simulink model "new1"  (R2025a)
settings: Solver=ode15s  StartTime=0.0  StopTime=10.0  RelTol=1e-3
undefined symbols (not defined in the file): g, Rs, Rsl, Rw, Ry, ShaftDamping, SolverSampleTime
libraries: fl_lib x44, nesl_utility x13, ee_lib x12, slpidlib x3, spsThreePhaseParallelRLCBranchLib x1, simrfV2elements x1, eePwmGeneratorTwoLevel x1, simulink x1, spsabctodq0Lib x1, spspowerguiLib x1
settings Model: SimulationMode=accelerator  Creator=maska  LastModifiedBy=maska

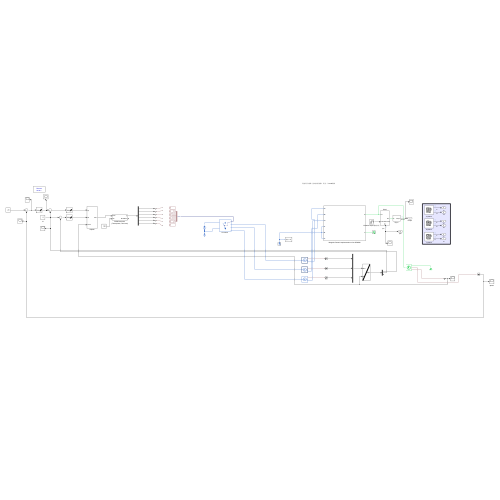
[thumbnail: Simulink's stored preview of the top-level diagram]
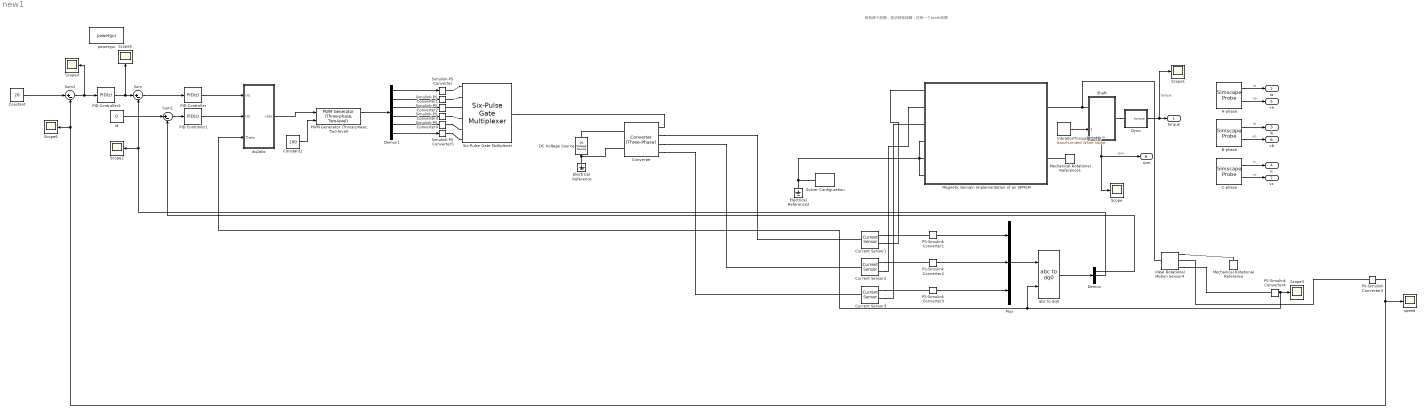
== system new1 ==
  note: 现有两个故障，扰动转矩故障，还有一个tooth故障
  A-phase : SimscapeProbe  BoundBlock=214  Variables="{\"i\":{\"Probing\":\"ON\"},\"n.v\":{\"Probing\":\"ON\"}}"
  B-phase : SimscapeProbe  BoundBlock=215  Variables="{\"i\":{\"Probing\":\"ON\"},\"n.v\":{\"Probing\":\"ON\"}}"
  C-phase : SimscapeProbe  BoundBlock=216  Variables="{\"i\":{\"Probing\":\"ON\"},\"n.v\":{\"Probing\":\"ON\"}}"
  Constant : Constant  Value=20
  Constant1 : Constant  Value=100
  Converter : ee_lib/Semiconductors & Converters/Converters/Converter (Three-Phase)  port_option=ee.enum.threePhasePort.expanded  fidelity_option=ee.enum.converters.fidelity.detailed  device_type=3  showThermalPort=false  K=0  Vth=0.5 V  Vgt=1 V  Vgt_off=-1 V  Ih=1 A  Vf=0.8 V  Ron=0.001 Ohm  Rds=0.001 Ohm  Goff=1e-5 1/Ohm  Eon_scalar=22.86e-3 J  Eoff_scalar=17.14e-3 J  Eoff_natural_commutation=10e-3 J  Voff=300 V  Iout_scalar=600 A  onCurrentMeasDelay=0 s  useCurrentFromPreviousCycle=false  useVoltageFromPreviousCycle=false  diode_param=2  diode_Vf=0.8 V  diode_Ron=0.001 Ohm  diode_Goff=1e-5 1/Ohm  diode_C=50 nF  diode_iRM=-235 A  diode_iF=300 A  diode_idot=-50 A/us  diode_trr_param=1  diode_trr_factor=3  diode_trr=15 us  diode_Qrr=1.5e+3 s*uA  diode_rec_loss_model=ee.enum.diode.reverseRecoveryModel.fixed  diode_ErecVal=0 J  diode_scaleWithIandV=false  diode_ErecMat=zeros(2, 3) J  diode_TjrecVec=[298.15, 398.15] K  diode_IfrecVec=[.1, 1, 10] A  diode_IrecVal=10 A  diode_VrecVal=10 V  diode_tFilter=1 / 1000 / 100 s  thermal_network_parameterization=ee.enum.thermalNetworkTopology.external  Rth=[.08, .5] K/W  Rth_Cauer=[.08, .1, .5] K/W  Rth_Foster=[.08, .14, .22, .16] K/W  thermal_mass_parameterization=ee.enum.thermalNetwork.timeconstant  thermal_mass=[.01, .5] J/K  thermal_mass_Cauer=[.01, .1, .5] J/K  thermal_mass_Foster=[.001, .005, .05, .5] J/K  thermal_time_constant=[.001, .2] s  thermal_time_constant_Cauer=[.001, .1, .2] s  thermal_time_constant_Foster=[7e-05, .0007, .01, .08] s  thermal_mass_initial_temperatures=[25, 25] degC  thermal_mass_initial_temperatures_Cauer=[25, 25, 25] degC  junction_thermal_mass=0.01 J/K  Tvec_initial_Foster=[25, 25, 25, 25] degC  snubber_type=0  Cs=1e-7 F  Rs=0.1 Ohm  Vce_loss=[0, 150, 300] V
      settings: InternalSimscapePortConfiguration="{\"Bottom\":[],\"Left\":[{\"id\":\"G\",\"label\":\"G\",\"type\":\"foundation.electrical.twelve_phase\"},{\"id\":\"a\",\"label\":\"a\",\"type\":\"foundation.electrical.electrical\"},{\"id\":\"b\",\"label\":\"b\",\"type\":\"foundation.electrical.electrical\"},{\"id\":\"c\",\"label\":\"c\",\"type\":\"foundation.electrical.electrical\"}],\"Right\":[{\"id\":\"p\",\"label\":\"+\",\"type\":\"foundation.electrical.electrical\"},{\"id\":\"n\",\"label\":\"-\",\"type\":\"foundation.electrical.electrical\"}],\"Top\":[]}"
  Current Sensor1 : fl_lib/Electrical/Electrical Sensors/Current Sensor
  Current Sensor2 : fl_lib/Electrical/Electrical Sensors/Current Sensor
  Current Sensor3 : fl_lib/Electrical/Electrical Sensors/Current Sensor
  DC Voltage Source : fl_lib/Electrical/Electrical Sources/DC Voltage Source  v0=750 V
  Demux : Demux  Outputs=3
  Demux1 : Demux  Outputs=6
  Dyno : Subsystem
  Electrical Reference : fl_lib/Electrical/Electrical Elements/Electrical Reference
  Electrical Reference2 : fl_lib/Electrical/Electrical Elements/Electrical Reference
  Ideal Rotational Motion Sensor4 : fl_lib/Mechanical/Mechanical Sensors/Ideal Rotational Motion Sensor  reference=foundation.enum.MeasurementReference.difference  acceleration_port=false  velocity_port=true  position_port=true  wrap_angle=false  offset=0 rad
  Magnetic Domain Implementation of an SPMSM : Subsystem
  Mechanical Rotational Reference : fl_lib/Mechanical/Rotational Elements/Mechanical Rotational Reference
  Mechanical Rotational Reference1 : fl_lib/Mechanical/Rotational Elements/Mechanical Rotational Reference
  Mux : Mux  Inputs=3
  PID Controller : slpidlib/PID Controller  Controller=PID  Form=Parallel  TimeDomain=Discrete-time  UseExternalTs=off  SampleTime=-1  IntegratorMethod=Forward Euler  FilterMethod=Forward Euler  ControllerParametersSource=internal  P=10  I=100  UseKiTs=off  D=0  UseExternalDerivativeSource=off  N=100  UseFilter=on  TunerSelectOption=Transfer Function Based (PID Tuner App)  InitialConditionSource=internal  InitialConditionForIntegrator=0  InitialConditionForFilter=0  DifferentiatorICPrevScaledInput=0  ExternalReset=none  TrackingMode=off  Kt=1  LimitOutput=on  SatLimitsSource=internal  UpperSaturationLimit=1000  LowerSaturationLimit=-1000  LinearizeAsGain=on  AntiWindupMode=none  Kb=1  LimitIntegrator=off  UpperIntegratorSaturationLimit=inf  LowerIntegratorSaturationLimit=-inf  POutMin=[]  POutMax=[]  IOutMin=[]  IOutMax=[]  DOutMin=[]  DOutMax=[]  NOutMin=[]  NOutMax=[]  SumOutMin=[]  SumOutMax=[]  SaturationOutMin=[]  SaturationOutMax=[]  PParamMin=[]  PParamMax=[]  IParamMin=[]  IParamMax=[]  DParamMin=[]  DParamMax=[]  NParamMin=[]  NParamMax=[]  KbParamMin=[]  KbParamMax=[]  KtParamMin=[]  KtParamMax=[]  KbOutMin=[]  KbOutMax=[]  KtOutMin=[]  KtOutMax=[]  IntegratorOutMin=[]  IntegratorOutMax=[]  FilterOutMin=[]  FilterOutMax=[]  SumI1OutMin=[]  SumI1OutMax=[]  SumI2OutMin=[]  SumI2OutMax=[]  SumI3OutMin=[]  SumI3OutMax=[]  SumI4OutMin=[]  SumI4OutMax=[]  SumDOutMin=[]  SumDOutMax=[]  DifferentiatorOutMin=[]  DifferentiatorOutMax=[]  FilterDiffOutCoefMin=[]  FilterDiffOutCoefMax=[]  ReciprocalOutMin=[]  ReciprocalOutMax=[]  SumDenOutMin=[]  SumDenOutMax=[]  SumNumOutMin=[]  SumNumOutMax=[]  DivideOutMin=[]  DivideOutMax=[]  UdiffTsProdOutMin=[]  UdiffTsProdOutMax=[]  NTsProdOutMin=[]  NTsProdOutMax=[]  UintegralTsProdOutMin=[]  UintegralTsProdOutMax=[]  UngainTsProdOutMin=[]  UngainTsProdOutMax=[]  ClampingZeroOutDataTypeStr=Inherit: Inherit via back propagation  ClampingZeroOutMin=[]  ClampingZeroOutMax=[]  FilterDenConstantOutDataTypeStr=Inherit: Inherit via back propagation  FilterDenConstantOutMin=[]  FilterDenConstantOutMax=[]  PCopyOutDataTypeStr=Inherit: Inherit via back propagation  PCopyOutMin=[]  PCopyOutMax=[]  NCopyOutDataTypeStr=Inherit: Inherit via back propagation  NCopyOutMin=[]  NCopyOutMax=[]  IntegratorContinuousStateAttributes=''  IntegratorStateMustResolveToSignalObject=off  IntegratorRTWStateStorageClass=Auto  FilterContinuousStateAttributes=''  FilterStateMustResolveToSignalObject=off  FilterRTWStateStorageClass=Auto  ParallelPVariant=InternalParameters  IdealPVariant=Disabled  IVariant=InternalParameters  DVariant=InternalParameters  IntegratorVariant=Discrete  SatVariant=Enabled  AWVariant=Passthrough  PCopyVariant=Disabled  TRVariant=Disabled  FdbkBlocksVariant=Forward  IdealPFdbkVariant=Disabled  SatFdbkVariant=Disabled  DerivativeFilterVariant=ForwardEulerFilter  NVariant=InternalParameters  NCopyVariant=Disabled  FilterICVariant=InternalICsFilter  IntegratorICVariant=InternalICs  ExternalResetVariant=Disabled  TRSumVariant=Passthrough  SumFdbkVariant=Disabled  SumVariant=Sum_PID  TsampFilterVariant=InternalTs  TsampNgainVariant=Passthrough  TsampIntegralVariant=Disabled_SignalSpec  ExternalSaturationOutDataTypeStr=Inherit: Same as second input  DerivativeSourceVariant=ErrorSignal  PreIntVariant=InternalPreInt
  PID Controller1 : slpidlib/PID Controller  Controller=PID  Form=Parallel  TimeDomain=Discrete-time  UseExternalTs=off  SampleTime=-1  IntegratorMethod=Forward Euler  FilterMethod=Forward Euler  ControllerParametersSource=internal  P=4  I=45  UseKiTs=off  D=0  UseExternalDerivativeSource=off  N=100  UseFilter=on  TunerSelectOption=Transfer Function Based (PID Tuner App)  InitialConditionSource=internal  InitialConditionForIntegrator=0  InitialConditionForFilter=0  DifferentiatorICPrevScaledInput=0  ExternalReset=none  TrackingMode=off  Kt=1  LimitOutput=on  SatLimitsSource=internal  UpperSaturationLimit=1000  LowerSaturationLimit=-1000  LinearizeAsGain=on  AntiWindupMode=none  Kb=1  LimitIntegrator=off  UpperIntegratorSaturationLimit=inf  LowerIntegratorSaturationLimit=-inf  POutMin=[]  POutMax=[]  IOutMin=[]  IOutMax=[]  DOutMin=[]  DOutMax=[]  NOutMin=[]  NOutMax=[]  SumOutMin=[]  SumOutMax=[]  SaturationOutMin=[]  SaturationOutMax=[]  PParamMin=[]  PParamMax=[]  IParamMin=[]  IParamMax=[]  DParamMin=[]  DParamMax=[]  NParamMin=[]  NParamMax=[]  KbParamMin=[]  KbParamMax=[]  KtParamMin=[]  KtParamMax=[]  KbOutMin=[]  KbOutMax=[]  KtOutMin=[]  KtOutMax=[]  IntegratorOutMin=[]  IntegratorOutMax=[]  FilterOutMin=[]  FilterOutMax=[]  SumI1OutMin=[]  SumI1OutMax=[]  SumI2OutMin=[]  SumI2OutMax=[]  SumI3OutMin=[]  SumI3OutMax=[]  SumI4OutMin=[]  SumI4OutMax=[]  SumDOutMin=[]  SumDOutMax=[]  DifferentiatorOutMin=[]  DifferentiatorOutMax=[]  FilterDiffOutCoefMin=[]  FilterDiffOutCoefMax=[]  ReciprocalOutMin=[]  ReciprocalOutMax=[]  SumDenOutMin=[]  SumDenOutMax=[]  SumNumOutMin=[]  SumNumOutMax=[]  DivideOutMin=[]  DivideOutMax=[]  UdiffTsProdOutMin=[]  UdiffTsProdOutMax=[]  NTsProdOutMin=[]  NTsProdOutMax=[]  UintegralTsProdOutMin=[]  UintegralTsProdOutMax=[]  UngainTsProdOutMin=[]  UngainTsProdOutMax=[]  ClampingZeroOutDataTypeStr=Inherit: Inherit via back propagation  ClampingZeroOutMin=[]  ClampingZeroOutMax=[]  FilterDenConstantOutDataTypeStr=Inherit: Inherit via back propagation  FilterDenConstantOutMin=[]  FilterDenConstantOutMax=[]  PCopyOutDataTypeStr=Inherit: Inherit via back propagation  PCopyOutMin=[]  PCopyOutMax=[]  NCopyOutDataTypeStr=Inherit: Inherit via back propagation  NCopyOutMin=[]  NCopyOutMax=[]  IntegratorContinuousStateAttributes=''  IntegratorStateMustResolveToSignalObject=off  IntegratorRTWStateStorageClass=Auto  FilterContinuousStateAttributes=''  FilterStateMustResolveToSignalObject=off  FilterRTWStateStorageClass=Auto  ParallelPVariant=InternalParameters  IdealPVariant=Disabled  IVariant=InternalParameters  DVariant=InternalParameters  IntegratorVariant=Discrete  SatVariant=Enabled  AWVariant=Passthrough  PCopyVariant=Disabled  TRVariant=Disabled  FdbkBlocksVariant=Forward  IdealPFdbkVariant=Disabled  SatFdbkVariant=Disabled  DerivativeFilterVariant=ForwardEulerFilter  NVariant=InternalParameters  NCopyVariant=Disabled  FilterICVariant=InternalICsFilter  IntegratorICVariant=InternalICs  ExternalResetVariant=Disabled  TRSumVariant=Passthrough  SumFdbkVariant=Disabled  SumVariant=Sum_PID  TsampFilterVariant=InternalTs  TsampNgainVariant=Passthrough  TsampIntegralVariant=Disabled_SignalSpec  ExternalSaturationOutDataTypeStr=Inherit: Same as second input  DerivativeSourceVariant=ErrorSignal  PreIntVariant=InternalPreInt
  PID Controller2 : slpidlib/PID Controller  Controller=PID  Form=Parallel  TimeDomain=Discrete-time  UseExternalTs=off  SampleTime=-1  IntegratorMethod=Forward Euler  FilterMethod=Forward Euler  ControllerParametersSource=internal  P=2.5  I=40  UseKiTs=off  D=0  UseExternalDerivativeSource=off  N=100  UseFilter=on  TunerSelectOption=Transfer Function Based (PID Tuner App)  InitialConditionSource=internal  InitialConditionForIntegrator=0  InitialConditionForFilter=0  DifferentiatorICPrevScaledInput=0  ExternalReset=none  TrackingMode=off  Kt=1  LimitOutput=on  SatLimitsSource=internal  UpperSaturationLimit=10000  LowerSaturationLimit=-10000  LinearizeAsGain=on  AntiWindupMode=none  Kb=1  LimitIntegrator=off  UpperIntegratorSaturationLimit=inf  LowerIntegratorSaturationLimit=-inf  POutMin=[]  POutMax=[]  IOutMin=[]  IOutMax=[]  DOutMin=[]  DOutMax=[]  NOutMin=[]  NOutMax=[]  SumOutMin=[]  SumOutMax=[]  SaturationOutMin=[]  SaturationOutMax=[]  PParamMin=[]  PParamMax=[]  IParamMin=[]  IParamMax=[]  DParamMin=[]  DParamMax=[]  NParamMin=[]  NParamMax=[]  KbParamMin=[]  KbParamMax=[]  KtParamMin=[]  KtParamMax=[]  KbOutMin=[]  KbOutMax=[]  KtOutMin=[]  KtOutMax=[]  IntegratorOutMin=[]  IntegratorOutMax=[]  FilterOutMin=[]  FilterOutMax=[]  SumI1OutMin=[]  SumI1OutMax=[]  SumI2OutMin=[]  SumI2OutMax=[]  SumI3OutMin=[]  SumI3OutMax=[]  SumI4OutMin=[]  SumI4OutMax=[]  SumDOutMin=[]  SumDOutMax=[]  DifferentiatorOutMin=[]  DifferentiatorOutMax=[]  FilterDiffOutCoefMin=[]  FilterDiffOutCoefMax=[]  ReciprocalOutMin=[]  ReciprocalOutMax=[]  SumDenOutMin=[]  SumDenOutMax=[]  SumNumOutMin=[]  SumNumOutMax=[]  DivideOutMin=[]  DivideOutMax=[]  UdiffTsProdOutMin=[]  UdiffTsProdOutMax=[]  NTsProdOutMin=[]  NTsProdOutMax=[]  UintegralTsProdOutMin=[]  UintegralTsProdOutMax=[]  UngainTsProdOutMin=[]  UngainTsProdOutMax=[]  ClampingZeroOutDataTypeStr=Inherit: Inherit via back propagation  ClampingZeroOutMin=[]  ClampingZeroOutMax=[]  FilterDenConstantOutDataTypeStr=Inherit: Inherit via back propagation  FilterDenConstantOutMin=[]  FilterDenConstantOutMax=[]  PCopyOutDataTypeStr=Inherit: Inherit via back propagation  PCopyOutMin=[]  PCopyOutMax=[]  NCopyOutDataTypeStr=Inherit: Inherit via back propagation  NCopyOutMin=[]  NCopyOutMax=[]  IntegratorContinuousStateAttributes=''  IntegratorStateMustResolveToSignalObject=off  IntegratorRTWStateStorageClass=Auto  FilterContinuousStateAttributes=''  FilterStateMustResolveToSignalObject=off  FilterRTWStateStorageClass=Auto  ParallelPVariant=InternalParameters  IdealPVariant=Disabled  IVariant=InternalParameters  DVariant=InternalParameters  IntegratorVariant=Discrete  SatVariant=Enabled  AWVariant=Passthrough  PCopyVariant=Disabled  TRVariant=Disabled  FdbkBlocksVariant=Forward  IdealPFdbkVariant=Disabled  SatFdbkVariant=Disabled  DerivativeFilterVariant=ForwardEulerFilter  NVariant=InternalParameters  NCopyVariant=Disabled  FilterICVariant=InternalICsFilter  IntegratorICVariant=InternalICs  ExternalResetVariant=Disabled  TRSumVariant=Passthrough  SumFdbkVariant=Disabled  SumVariant=Sum_PID  TsampFilterVariant=InternalTs  TsampNgainVariant=Passthrough  TsampIntegralVariant=Disabled_SignalSpec  ExternalSaturationOutDataTypeStr=Inherit: Same as second input  DerivativeSourceVariant=ErrorSignal  PreIntVariant=InternalPreInt
  PS-Simulink Converter{1..5} (5 alike) : nesl_utility/PS-Simulink Converter  PhysicalDomain=network_engine_domain  SubClassName=ps_output  LeftPortType=input  RightPortType=output  PseudoPeriodic=off  Frequencies=[]  VectorFormat=inherit  Unit=inherit  AffineConversion=off
  "PWM Generator (Three-phase, Two-level)" : eePwmGeneratorTwoLevel/PWM Generator (Three-phase, Two-level)  PWMMode=Continuous PWM (CPWM)  CPWMMode=SPWM: sinusoidal PWM  DPWMMode=60 DPWM: 60 degree discontinuous PWM  fsw=1e3  Ts=2e-6
      settings: LibrarySourceBlock=|
      | ee_sl_lib/Pulse Width
      | Modulation/PWM Generator
      | (Three-phase, Two-level)
  Scope{,1..6} (7 alike) : Scope
      Scope settings: ActiveDisplayYMinimum=5.9889874068411224  ActiveDisplayYMaximum=16.410945963930487
      Scope1 settings: ActiveDisplayYMinimum=-17672.734869868404  ActiveDisplayYMaximum=1963.7070418694955  DataLoggingVariableName=ScopeData2
      Scope2 settings: ActiveDisplayYMinimum=-0.416473738906253  ActiveDisplayYMaximum=0.436398147050316  YLabel=скорость  DataLoggingVariableName=ScopeData5
      Scope3 settings: ActiveDisplayYMinimum=-20.943872983065386  ActiveDisplayYMaximum=188.49485684758849  DataLoggingVariableName=ScopeData3
      Scope4 settings: ActiveDisplayYMinimum=2.2678285118136117  ActiveDisplayYMaximum=20.092232680750982  YLabel=скорость  DataLoggingVariableName=ScopeData8
      Scope5 settings: ActiveDisplayYMinimum=-203.76901912599916  ActiveDisplayYMaximum=1942.3454210939431  YLabel=скорость  DataLoggingVariableName=ScopeData9
      Scope6 settings: ActiveDisplayYMinimum=-2.0472362485662443  ActiveDisplayYMaximum=18.4251262370962  YLabel=скорость  DataLoggingVariableName=ScopeData6
  Shaft : Subsystem
      settings: PortSchema="{\"entries\":[{\"content\":{\"sides\":[{\"content\":{\"connectorIds\":[\"In1\",\"LConn1\"]},\"type\":\"ConnectorPlacement.EquallySpacedRectSide\",\"uuid\":\"d15f0b0a-376f-42bd-94fa-6b80795b7e9e\"},{\"content\":{\"connectorIds\":[\"RConn1\"],\"side\":\"RIGHT\"},\"type\":\"ConnectorPlacement.EquallySpacedRectSide\",\"uuid\":\"1c10d066-ee05-4c09-9add-16f0039017c8\"},{\"content\":{\"connectorIds\":[\"Out1\"],\"side\":\"TOP\"},\"type\":\"ConnectorPlacement.EquallySpacedRectSide\",\"uuid\":\"1eb1d482-04bc-4375-925a-bb39b5ad5755\"},{\"content\":{\"side\":\"BOTTOM\"},\"type\":\"ConnectorPlacement.EquallySpacedRectSide\",\"uuid\":\"41e2e734-a35c-40f7-83b7-7f9932e1f2da\"}]},\"type\":\"ConnectorPlacement.EquallySpacedConnector\",\"uuid\":\"850c0d3a-bd0e-4af5-8553-9696ca3cdee9\"}],\"packageUris\":[\"http://schema.mathworks.com/mf0/Connector/R2020b\"],\"version\":\"1.0\"}"
  Simulink-PS Converter{,1..5} (6 alike) : nesl_utility/Simulink-PS Converter  PhysicalDomain=network_engine_domain  SubClassName=ps_input  LeftPortType=input  RightPortType=output  PseudoPeriodic=off  Frequencies=[]  NoiseDistribution=none  NoiseParameters=[]  Unit=1  AffineConversion=off  FilteringAndDerivatives=provide  SimscapeFilterOrder=1  InputFilterTimeConstant=0.001  UdotUserProvided=0
  Six-Pulse Gate Multiplexer : ee_lib/Semiconductors & Converters/Converters/Six-Pulse Gate Multiplexer  port_option=ee.enum.controlport.ps
  Solver Configuration : nesl_utility/Solver Configuration  PhysicalDomain=network_engine_domain  SubClassName=solver  LeftPortType=input  RightPortType=generic  Tones=[]  Harmonics=[]  SimulateNoise=off  Profile=off  UseLocalSampling=off  EnableSwitchedLinearOptims=on  FrequencyDomain=off  UseCCode=off  RelTol=0.001  AbsTol=1e-06  MinStep=1e-09  ToWorkspace=off  RevertToSquareIcSolve=off  NumHomotopyIterations=100  PhasorMode=off  PhasorModeNumHarmonics=1  ConsistencySolver=NEWTON_FTOL  IndexReductionMethod=DerivativeReplacement  DoDC=off  ResidualTolerance=1e-09  ConsistencyTolSource=GLOBAL  ConsistencyAbsTol=0.001  ConsistencyRelTol=0.001  ConsistencyTolFactor=0.001  UseLocalSolver=on  LocalSolverChoice=NE_BACKWARD_EULER_ADVANCER  ResolveIndetEquations=on  FunctionEvalNumThread=1  LocalSolverSampleTime=SolverSampleTime  DoFixedCost=off  MaxNonlinIter=3  MaxModeIter=2  ComputeImpulses=off  ImpulseIterations=1  LinearAlgebra=auto  LinearAlgebraNumThread=0  EquationFormulation=NE_TIME_EF  DelaysMemoryBudget=1024  AutomaticFiltering=on  FilteringTimeConstant=0.001  PartitionStorageMethod=AS_NEEDED  PartitionMemoryBudget=1024  PartitionMethod=ROBUST  MultibodyUseLocalSolver=off  MultibodyLocalSolverChoice=ODE1  MultibodyLocalSolverSampleTime=0.001
  Sum : Sum  Inputs=|+-
  Sum1 : Sum  Inputs=|+-
  Sum2 : Sum  Inputs=|+-
  VibrationTorque震动转矩 : simulink/Sources/Band-Limited White Noise  Cov=VibrationNoisePower  Ts=SolverSampleTime  seed=[23341]
  abc to dq0 : spsabctodq0Lib/abc to dq0  Alignment=90 degrees behind phase A axis
  dq2abc : Subsystem
  id : Constant  Value=0
  powergui : spspowerguiLib/powergui  Priority=1  SimulationMode=Discrete  SampleTime=2e-6  frequency=60  Iterations=50  frequencyindice=0  Pbase=100e6  ErrMax=1e-4  UnitsV=kV  UnitsW=MW  buscounter=0  FunctionMessages=off  echomessages=off  EnableUseOfTLC=off  CurrentSourceSwitches=off  DisableSnubberDevices=off  DisableRonSwitches=off  DisableVfSwitches=off  DisplayEquations=off  AutomaticDiscreteSolvers=off  SolverType=Tustin/Backward Euler (TBE)  Interpol=off  ExternalGateDelay=off  methode=off  Ts=100  x0status=blocks  SPID=on  SwTol=0  HookPort=off  NonlinearTolerance=1e-4  nMaxIteration=100  ContinueOnMaxIteration=off  RestoreLinks=warning  ResistiveCurrentMeasurement=off  Frange=[0:2:500]  Ylog=off  Xlog=on  ShowGrid=off  save=off  variable=ZData  structure=0  ZoomFFT=off  StartTime=0.0  cycles=1  DisplayStyle=1  fundamental=60  FreqAxis=off  MaxFrequency=1000  frequencyindicesteady=1  RmsSteady=1  display=off
  speed : Scope
      settings: ActiveDisplayYMinimum=15.541713214540213  ActiveDisplayYMaximum=15.760330288068594  DataLoggingVariableName=ScopeData7
  torque : Outport
  ia : Outport  Port=2
  ib : Outport  Port=3
  ic : Outport  Port=4
  va : Outport  Port=5
  vb : Outport  Port=6
  vc : Outport  Port=7
  rpm : Outport  Port=8
  wires:
  VibrationTorque震动转矩/1 -> Shaft/1(PerturbationTorque)
  Dyno/1(torque) -> Scope1/1, torque/1  "torque"
  B-phase/2 -> vb/1  "vb"
  C-phase/2 -> vc/1  "vc"
  A-phase/1 -> ia/1  "ia"
  Shaft/1(rpm) -> Scope/1, rpm/1  "rpm"
  C-phase/1 -> ic/1  "ic"
  B-phase/1 -> ib/1  "ib"
  A-phase/2 -> va/1  "va"
  Sum2/1 -> Scope4/1, PID Controller2/1
  PID Controller2/1 -> Sum/1, Scope5/1
  Constant/1 -> Sum2/1
  id/1 -> Sum1/1
  Sum1/1 -> PID Controller1/1
  Demux/1 -> Sum1/2
  PS-Simulink Converter5/1 -> speed/1, Sum2/2, Scope6/1
  Demux/2 -> Scope2/1, Sum/2
  PS-Simulink Converter4/1 -> dq2abc/3(Theta), abc to dq0/2, Scope3/1
  PID Controller/1 -> dq2abc/1(Uq)
  PID Controller1/1 -> dq2abc/2(Ud)
  Sum/1 -> PID Controller/1
  PS-Simulink Converter3/1 -> Mux/3
  PS-Simulink Converter2/1 -> Mux/2
  PS-Simulink Converter1/1 -> Mux/1
  Mux/1 -> abc to dq0/1
  abc to dq0/1 -> Demux/1
  Constant1/1 -> "PWM Generator (Three-phase, Two-level)"/2
  dq2abc/1(vabc) -> "PWM Generator (Three-phase, Two-level)"/1
  "PWM Generator (Three-phase, Two-level)"/1 -> Demux1/1
  Demux1/6 -> Simulink-PS Converter5/1
  Demux1/5 -> Simulink-PS Converter4/1
  Demux1/2 -> Simulink-PS Converter1/1
  Demux1/1 -> Simulink-PS Converter/1
  Demux1/4 -> Simulink-PS Converter3/1
  Demux1/3 -> Simulink-PS Converter2/1
  connections:
  Solver Configuration/RConn1 -- Electrical Reference2/LConn1 -- Magnetic Domain Implementation of an SPMSM/LConn4 -- Magnetic Domain Implementation of an SPMSM/LConn5 -- Magnetic Domain Implementation of an SPMSM/LConn6
  Ideal Rotational Motion Sensor4/LConn1 -- Magnetic Domain Implementation of an SPMSM/RConn1 -- Shaft/LConn1
  Shaft/RConn1 -- Dyno/LConn1
  Electrical Reference/LConn1 -- Converter/RConn2 -- DC Voltage Source/RConn1
  DC Voltage Source/LConn1 -- Converter/RConn1
  Current Sensor3/RConn2 -- Magnetic Domain Implementation of an SPMSM/LConn3
  Current Sensor2/RConn2 -- Magnetic Domain Implementation of an SPMSM/LConn2
  Current Sensor1/RConn2 -- Magnetic Domain Implementation of an SPMSM/LConn1
  Converter/LConn2 -- Current Sensor1/LConn1
  Converter/LConn3 -- Current Sensor2/LConn1
  Converter/LConn4 -- Current Sensor3/LConn1
  Current Sensor1/RConn1 -- PS-Simulink Converter1/LConn1
  Current Sensor2/RConn1 -- PS-Simulink Converter2/LConn1
  Current Sensor3/RConn1 -- PS-Simulink Converter3/LConn1
  Mechanical Rotational Reference1/LConn1 -- Magnetic Domain Implementation of an SPMSM/RConn2
  Ideal Rotational Motion Sensor4/RConn1 -- Mechanical Rotational Reference/LConn1
  Ideal Rotational Motion Sensor4/RConn3 -- PS-Simulink Converter4/LConn1
  PS-Simulink Converter5/LConn1 -- Ideal Rotational Motion Sensor4/RConn2
  Simulink-PS Converter5/RConn1 -- Six-Pulse Gate Multiplexer/LConn6
  Simulink-PS Converter3/RConn1 -- Six-Pulse Gate Multiplexer/LConn4
  Simulink-PS Converter/RConn1 -- Six-Pulse Gate Multiplexer/LConn1
  Simulink-PS Converter4/RConn1 -- Six-Pulse Gate Multiplexer/LConn5
  Simulink-PS Converter2/RConn1 -- Six-Pulse Gate Multiplexer/LConn3
  Simulink-PS Converter1/RConn1 -- Six-Pulse Gate Multiplexer/LConn2
  Six-Pulse Gate Multiplexer/RConn1 -- Converter/LConn1

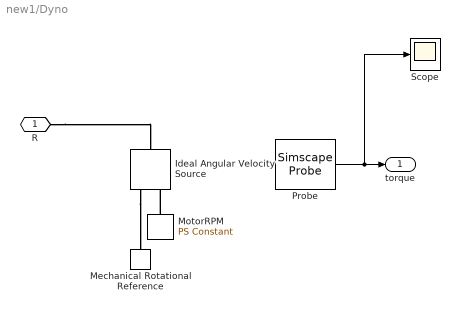
== system new1/Dyno ==
  Ideal Angular Velocity Source : fl_lib/Mechanical/Mechanical Sources/Ideal Angular Velocity Source
  Mechanical Rotational Reference : fl_lib/Mechanical/Rotational Elements/Mechanical Rotational Reference
  MotorRPM : fl_lib/Physical Signals/Sources/PS Constant  constant=motorRPM rpm
  Probe : SimscapeProbe  BoundBlock=148  Variables="{\"t\":{\"Probing\":\"ON\"}}"
  Scope : Scope
      settings: ActiveDisplayYMinimum=-17672.741352339104  ActiveDisplayYMaximum=1963.7653841058097
  R : PMIOPort  Side=Left
  torque : Outport
  wires:
  Probe/1 -> Scope/1, torque/1
  connections:
  MotorRPM/RConn1 -- Ideal Angular Velocity Source/RConn1
  Ideal Angular Velocity Source/RConn2 -- Mechanical Rotational Reference/LConn1
  R/RConn1 -- Ideal Angular Velocity Source/LConn1

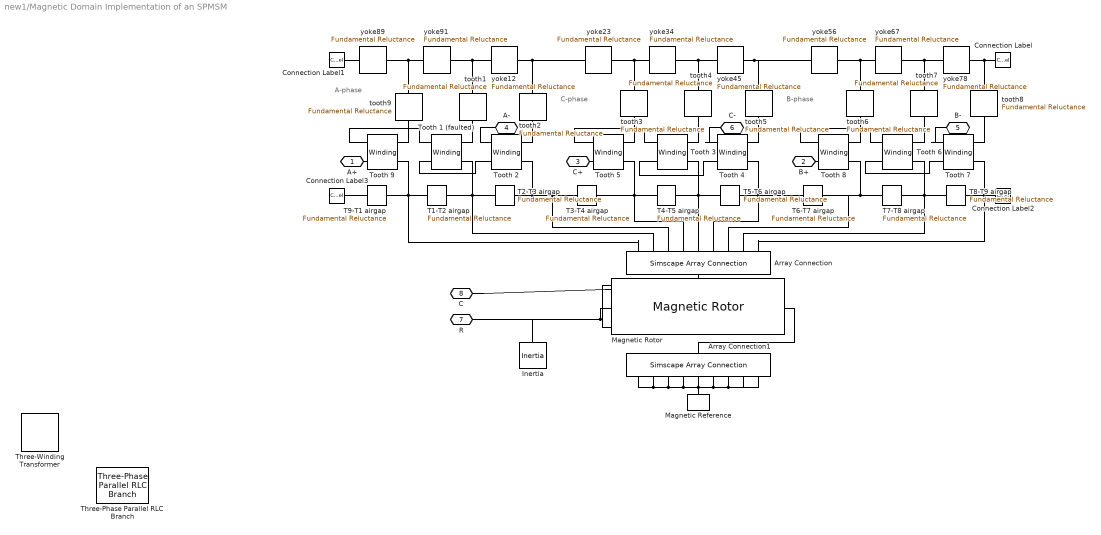
== system new1/Magnetic Domain Implementation of an SPMSM ==
  note: A-phase
  note: C-phase
  note: B-phase
  Array Connection : SimscapeArrayConnection  Domain=foundation.magnetic.magnetic  NumScalarElements=9
  Array Connection1 : SimscapeArrayConnection  Domain=foundation.magnetic.magnetic  NumScalarElements=9
  Connection Label : ConnectionLabel  Label=Y
  Connection Label1 : ConnectionLabel  Label=Y
  Connection Label2 : ConnectionLabel  Label=SL
  Connection Label3 : ConnectionLabel  Label=SL
  Inertia : fl_lib/Mechanical/Rotational Elements/Inertia  inertia=J kg*m^2  num_ports=foundation.enum.numPorts2.one  w_specify=on  w_priority=None  w=0 rad/s  w_nominal_specify=off  w_nominal_value=1  w_nominal_unit=rad/s  t_specify=off  t_priority=High  t=0 N*m  t_nominal_specify=off  t_nominal_value=1  t_nominal_unit=N*m
  Magnetic Reference : fl_lib/Magnetic/Magnetic Elements/Magnetic Reference
      settings: InternalSimscapePortConfiguration="{\"Bottom\":[],\"Left\":[{\"id\":\"M\",\"label\":\"\",\"type\":\"foundation.magnetic.magnetic\"}],\"Right\":[],\"Top\":[]}"
  Magnetic Rotor : ee_lib/Electromechanical/Magnetic Rotor  Nr=Npp  Ns=Ns  B0=B0 T  lm=lm mm  mur=1.05  g=g mm  r=r mm  l=l mm
      settings: InternalSimscapePortConfiguration="{\"Bottom\":[{\"id\":\"S\",\"label\":\"S\",\"type\":\"foundation.magnetic.magnetic\"}],\"Left\":[{\"id\":\"C\",\"label\":\"C\",\"type\":\"foundation.mechanical.rotational.rotational\"},{\"id\":\"R\",\"label\":\"R\",\"type\":\"foundation.mechanical.rotational.rotational\"}],\"Right\":[],\"Top\":[{\"id\":\"N\",\"label\":\"N\",\"type\":\"foundation.magnetic.magnetic\"}]}"
  T1-T2 airgap : fl_lib/Magnetic/Magnetic Elements/Fundamental Reluctance  R=Rsl 1/H  phi_specify=off  phi_priority=None  phi=0 Wb  phi_nominal_specify=off  phi_nominal_value=1  phi_nominal_unit=Wb  mmf_specify=off  mmf_priority=None  mmf=0 A  mmf_nominal_specify=off  mmf_nominal_value=1  mmf_nominal_unit=A
      settings: InternalSimscapePortConfiguration="{\"Bottom\":[],\"Left\":[{\"id\":\"N\",\"label\":\"N\",\"type\":\"foundation.magnetic.magnetic\"}],\"Right\":[{\"id\":\"S\",\"label\":\"S\",\"type\":\"foundation.magnetic.magnetic\"}],\"Top\":[]}"
  T2-T3 airgap : fl_lib/Magnetic/Magnetic Elements/Fundamental Reluctance  R=Rsl 1/H  phi_specify=off  phi_priority=None  phi=0 Wb  phi_nominal_specify=off  phi_nominal_value=1  phi_nominal_unit=Wb  mmf_specify=off  mmf_priority=None  mmf=0 A  mmf_nominal_specify=off  mmf_nominal_value=1  mmf_nominal_unit=A
      settings: InternalSimscapePortConfiguration="{\"Bottom\":[],\"Left\":[{\"id\":\"N\",\"label\":\"N\",\"type\":\"foundation.magnetic.magnetic\"}],\"Right\":[{\"id\":\"S\",\"label\":\"S\",\"type\":\"foundation.magnetic.magnetic\"}],\"Top\":[]}"
  T3-T4 airgap : fl_lib/Magnetic/Magnetic Elements/Fundamental Reluctance  R=Rsl 1/H  phi_specify=off  phi_priority=None  phi=0 Wb  phi_nominal_specify=off  phi_nominal_value=1  phi_nominal_unit=Wb  mmf_specify=off  mmf_priority=None  mmf=0 A  mmf_nominal_specify=off  mmf_nominal_value=1  mmf_nominal_unit=A
      settings: InternalSimscapePortConfiguration="{\"Bottom\":[],\"Left\":[{\"id\":\"N\",\"label\":\"N\",\"type\":\"foundation.magnetic.magnetic\"}],\"Right\":[{\"id\":\"S\",\"label\":\"S\",\"type\":\"foundation.magnetic.magnetic\"}],\"Top\":[]}"
  T4-T5 airgap : fl_lib/Magnetic/Magnetic Elements/Fundamental Reluctance  R=Rsl 1/H  phi_specify=off  phi_priority=None  phi=0 Wb  phi_nominal_specify=off  phi_nominal_value=1  phi_nominal_unit=Wb  mmf_specify=off  mmf_priority=None  mmf=0 A  mmf_nominal_specify=off  mmf_nominal_value=1  mmf_nominal_unit=A
      settings: InternalSimscapePortConfiguration="{\"Bottom\":[],\"Left\":[{\"id\":\"N\",\"label\":\"N\",\"type\":\"foundation.magnetic.magnetic\"}],\"Right\":[{\"id\":\"S\",\"label\":\"S\",\"type\":\"foundation.magnetic.magnetic\"}],\"Top\":[]}"
  T5-T6 airgap : fl_lib/Magnetic/Magnetic Elements/Fundamental Reluctance  R=Rsl 1/H  phi_specify=off  phi_priority=None  phi=0 Wb  phi_nominal_specify=off  phi_nominal_value=1  phi_nominal_unit=Wb  mmf_specify=off  mmf_priority=None  mmf=0 A  mmf_nominal_specify=off  mmf_nominal_value=1  mmf_nominal_unit=A
      settings: InternalSimscapePortConfiguration="{\"Bottom\":[],\"Left\":[{\"id\":\"N\",\"label\":\"N\",\"type\":\"foundation.magnetic.magnetic\"}],\"Right\":[{\"id\":\"S\",\"label\":\"S\",\"type\":\"foundation.magnetic.magnetic\"}],\"Top\":[]}"
  T6-T7 airgap : fl_lib/Magnetic/Magnetic Elements/Fundamental Reluctance  R=Rsl 1/H  phi_specify=off  phi_priority=None  phi=0 Wb  phi_nominal_specify=off  phi_nominal_value=1  phi_nominal_unit=Wb  mmf_specify=off  mmf_priority=None  mmf=0 A  mmf_nominal_specify=off  mmf_nominal_value=1  mmf_nominal_unit=A
      settings: InternalSimscapePortConfiguration="{\"Bottom\":[],\"Left\":[{\"id\":\"N\",\"label\":\"N\",\"type\":\"foundation.magnetic.magnetic\"}],\"Right\":[{\"id\":\"S\",\"label\":\"S\",\"type\":\"foundation.magnetic.magnetic\"}],\"Top\":[]}"
  T7-T8 airgap : fl_lib/Magnetic/Magnetic Elements/Fundamental Reluctance  R=Rsl 1/H  phi_specify=off  phi_priority=None  phi=0 Wb  phi_nominal_specify=off  phi_nominal_value=1  phi_nominal_unit=Wb  mmf_specify=off  mmf_priority=None  mmf=0 A  mmf_nominal_specify=off  mmf_nominal_value=1  mmf_nominal_unit=A
      settings: InternalSimscapePortConfiguration="{\"Bottom\":[],\"Left\":[{\"id\":\"N\",\"label\":\"N\",\"type\":\"foundation.magnetic.magnetic\"}],\"Right\":[{\"id\":\"S\",\"label\":\"S\",\"type\":\"foundation.magnetic.magnetic\"}],\"Top\":[]}"
  T8-T9 airgap : fl_lib/Magnetic/Magnetic Elements/Fundamental Reluctance  R=Rsl 1/H  phi_specify=off  phi_priority=None  phi=0 Wb  phi_nominal_specify=off  phi_nominal_value=1  phi_nominal_unit=Wb  mmf_specify=off  mmf_priority=None  mmf=0 A  mmf_nominal_specify=off  mmf_nominal_value=1  mmf_nominal_unit=A
      settings: InternalSimscapePortConfiguration="{\"Bottom\":[],\"Left\":[{\"id\":\"N\",\"label\":\"N\",\"type\":\"foundation.magnetic.magnetic\"}],\"Right\":[{\"id\":\"S\",\"label\":\"S\",\"type\":\"foundation.magnetic.magnetic\"}],\"Top\":[]}"
  T9-T1 airgap : fl_lib/Magnetic/Magnetic Elements/Fundamental Reluctance  R=Rsl 1/H  phi_specify=off  phi_priority=None  phi=0 Wb  phi_nominal_specify=off  phi_nominal_value=1  phi_nominal_unit=Wb  mmf_specify=off  mmf_priority=None  mmf=0 A  mmf_nominal_specify=off  mmf_nominal_value=1  mmf_nominal_unit=A
      settings: InternalSimscapePortConfiguration="{\"Bottom\":[],\"Left\":[{\"id\":\"N\",\"label\":\"N\",\"type\":\"foundation.magnetic.magnetic\"}],\"Right\":[{\"id\":\"S\",\"label\":\"S\",\"type\":\"foundation.magnetic.magnetic\"}],\"Top\":[]}"
  Three-Phase Parallel RLC Branch : spsThreePhaseParallelRLCBranchLib/Three-Phase Parallel RLC Branch  LConnTagsString=A|B|C  RConnTagsString=A|B|C  BranchType=RLC  Resistance=1  Inductance=1e-3  Capacitance=1e-6  Measurements=None
  Three-Winding Transformer : simrfV2elements/Three-Winding Transformer  classname=three_winding_transformer  L1=1e-6 H  L2=1e-6 H  L3=1e-6 H  K12=0.9  K13=0.9  K23=0.9
  Tooth 1 (faulted) : ee_lib/Passive/Winding  Nw=Nws  Rw=Rw/3 Ohm  Rl=inf 1/H  Gw=gWinding 1/Ohm  thermalPort=simscape.enum.thermaleffects.omit  alpha=3.93e-3 1/K  Tmeas=25 degC  winding_thermal_mass=100 J/K  T_specify=off  T_priority=None  T=25 degC  T_nominal_specify=off  T_nominal_value=1  T_nominal_unit=degC  i_specify=off  i_priority=None  i=0 A  i_nominal_specify=off  i_nominal_value=1  i_nominal_unit=A  v_specify=off  v_priority=High  v=0 V  v_nominal_specify=off  v_nominal_value=1  v_nominal_unit=V  phi_specify=off  phi_priority=None  phi=0 Wb  phi_nominal_specify=off  phi_nominal_value=1  phi_nominal_unit=Wb  iterm_p_specify=off  iterm_p_priority=None  iterm_p=0 A  iterm_p_nominal_specify=off  iterm_p_nominal_value=1  iterm_p_nominal_unit=A  iterm_n_specify=off  iterm_n_priority=None  iterm_n=0 A  iterm_n_nominal_specify=off  iterm_n_nominal_value=1  iterm_n_nominal_unit=A  power_dissipated_specify=off  power_dissipated_priority=None  power_dissipated=0 W  power_dissipated_nominal_specify=off  power_dissipated_nominal_value=1  power_dissipated_nominal_unit=W
      settings: InternalSimscapePortConfiguration="{\"Bottom\":[],\"Left\":[{\"id\":\"p\",\"label\":\"+\",\"type\":\"foundation.electrical.electrical\"},{\"id\":\"n\",\"label\":\"-\",\"type\":\"foundation.electrical.electrical\"}],\"Right\":[{\"id\":\"N\",\"label\":\"N\",\"type\":\"foundation.magnetic.magnetic\"},{\"id\":\"S\",\"label\":\"S\",\"type\":\"foundation.magnetic.magnetic\"}],\"Top\":[]}"
  Tooth {2..9} (8 alike) : ee_lib/Passive/Winding  Nw=Nws  Rw=Rw/3 Ohm  Rl=inf 1/H  Gw=gWinding 1/Ohm  thermalPort=simscape.enum.thermaleffects.omit  alpha=3.93e-3 1/K  Tmeas=25 degC  winding_thermal_mass=100 J/K  T_specify=off  T_priority=None  T=25 degC  T_nominal_specify=off  T_nominal_value=1  T_nominal_unit=degC  i_specify=off  i_priority=None  i=0 A  i_nominal_specify=off  i_nominal_value=1  i_nominal_unit=A  v_specify=off  v_priority=None  v=0 V  v_nominal_specify=off  v_nominal_value=1  v_nominal_unit=V  phi_specify=off  phi_priority=None  phi=0 Wb  phi_nominal_specify=off  phi_nominal_value=1  phi_nominal_unit=Wb  iterm_p_specify=off  iterm_p_priority=None  iterm_p=0 A  iterm_p_nominal_specify=off  iterm_p_nominal_value=1  iterm_p_nominal_unit=A  iterm_n_specify=off  iterm_n_priority=None  iterm_n=0 A  iterm_n_nominal_specify=off  iterm_n_nominal_value=1  iterm_n_nominal_unit=A  power_dissipated_specify=off  power_dissipated_priority=None  power_dissipated=0 W  power_dissipated_nominal_specify=off  power_dissipated_nominal_value=1  power_dissipated_nominal_unit=W
      settings: InternalSimscapePortConfiguration="{\"Bottom\":[],\"Left\":[{\"id\":\"p\",\"label\":\"+\",\"type\":\"foundation.electrical.electrical\"},{\"id\":\"n\",\"label\":\"-\",\"type\":\"foundation.electrical.electrical\"}],\"Right\":[{\"id\":\"N\",\"label\":\"N\",\"type\":\"foundation.magnetic.magnetic\"},{\"id\":\"S\",\"label\":\"S\",\"type\":\"foundation.magnetic.magnetic\"}],\"Top\":[]}"
  tooth{1..9} (9 alike) : fl_lib/Magnetic/Magnetic Elements/Fundamental Reluctance  R=Rs 1/H  phi_specify=off  phi_priority=None  phi=0 Wb  phi_nominal_specify=off  phi_nominal_value=1  phi_nominal_unit=Wb  mmf_specify=off  mmf_priority=None  mmf=0 A  mmf_nominal_specify=off  mmf_nominal_value=1  mmf_nominal_unit=A
      settings: InternalSimscapePortConfiguration="{\"Bottom\":[],\"Left\":[{\"id\":\"N\",\"label\":\"N\",\"type\":\"foundation.magnetic.magnetic\"}],\"Right\":[{\"id\":\"S\",\"label\":\"S\",\"type\":\"foundation.magnetic.magnetic\"}],\"Top\":[]}"
  yoke{12,23,34,45,56,67,78,89,91} (9 alike) : fl_lib/Magnetic/Magnetic Elements/Fundamental Reluctance  R=Ry 1/H  phi_specify=off  phi_priority=None  phi=0 Wb  phi_nominal_specify=off  phi_nominal_value=1  phi_nominal_unit=Wb  mmf_specify=off  mmf_priority=None  mmf=0 A  mmf_nominal_specify=off  mmf_nominal_value=1  mmf_nominal_unit=A
      settings: InternalSimscapePortConfiguration="{\"Bottom\":[],\"Left\":[{\"id\":\"N\",\"label\":\"N\",\"type\":\"foundation.magnetic.magnetic\"}],\"Right\":[{\"id\":\"S\",\"label\":\"S\",\"type\":\"foundation.magnetic.magnetic\"}],\"Top\":[]}"
  A+ : PMIOPort  Side=Left
  B+ : PMIOPort  Port=2  Side=Left
  C+ : PMIOPort  Port=3  Side=Left
  A- : PMIOPort  Port=4  Side=Left
  B- : PMIOPort  Port=5  Side=Left
  C- : PMIOPort  Port=6  Side=Left
  R : PMIOPort  Port=7  Side=Right
  C : PMIOPort  Port=8  Side=Right
  connections:
  yoke91/RConn1 -- yoke12/LConn1 -- tooth1/LConn1
  Tooth 1 (faulted)/RConn2 -- Array Connection/LConn2 -- T2-T3 airgap/LConn1 -- T1-T2 airgap/RConn1
  T3-T4 airgap/LConn1 -- Array Connection/LConn3 -- Tooth 2/RConn2 -- T2-T3 airgap/RConn1
  Tooth 2/RConn1 -- tooth2/RConn1
  yoke91/LConn1 -- yoke89/RConn1 -- tooth9/LConn1
  yoke89/LConn1 -- Connection Label1/LConn1
  T9-T1 airgap/LConn1 -- Connection Label3/LConn1
  Tooth 9/LConn2 -- A+/RConn1
  Tooth 9/LConn1 -- Tooth 1 (faulted)/LConn1
  Tooth 1 (faulted)/LConn2 -- Tooth 2/LConn2
  Tooth 2/LConn1 -- A-/RConn1
  Tooth 9/RConn2 -- Array Connection/LConn1 -- T9-T1 airgap/RConn1 -- T1-T2 airgap/LConn1
  yoke45/LConn1 -- yoke34/RConn1 -- tooth4/LConn1
  Tooth 3/RConn2 -- Array Connection/LConn5 -- T5-T6 airgap/LConn1 -- T4-T5 airgap/RConn1
  T6-T7 airgap/LConn1 -- Array Connection/LConn6 -- T5-T6 airgap/RConn1 -- Tooth 4/RConn2
  yoke34/LConn1 -- yoke23/RConn1 -- tooth3/LConn1
  Magnetic Rotor/LConn2 -- Inertia/LConn1 -- R/RConn1
  Tooth 5/RConn2 -- Array Connection/LConn4 -- T3-T4 airgap/RConn1 -- T4-T5 airgap/LConn1
  yoke45/RConn1 -- yoke56/LConn1 -- tooth5/LConn1
  Tooth 5/LConn2 -- C+/RConn1
  Tooth 3/LConn2 -- Tooth 4/LConn2
  Tooth 5/LConn1 -- Tooth 3/LConn1
  Tooth 4/LConn1 -- C-/RConn1
  yoke78/LConn1 -- yoke67/RConn1 -- tooth7/LConn1
  Tooth 6/RConn2 -- Array Connection/LConn8 -- T8-T9 airgap/LConn1 -- T7-T8 airgap/RConn1
  T8-T9 airgap/RConn1 -- Array Connection/LConn9 -- Connection Label2/LConn1 -- Tooth 7/RConn2
  yoke67/LConn1 -- yoke56/RConn1 -- tooth6/LConn1
  Tooth 8/RConn2 -- Array Connection/LConn7 -- T6-T7 airgap/RConn1 -- T7-T8 airgap/LConn1
  C/RConn1 -- Magnetic Rotor/LConn1
  tooth8/LConn1 -- yoke78/RConn1 -- Connection Label/LConn1
  Tooth 8/LConn2 -- B+/RConn1
  Tooth 8/LConn1 -- Tooth 6/LConn1
  Tooth 6/LConn2 -- Tooth 7/LConn2
  Tooth 7/LConn1 -- B-/RConn1
  Tooth 1 (faulted)/RConn1 -- tooth1/RConn1
  yoke23/LConn1 -- tooth2/LConn1 -- yoke12/RConn1
  Tooth 5/RConn1 -- tooth3/RConn1
  Tooth 3/RConn1 -- tooth4/RConn1
  Tooth 4/RConn1 -- tooth5/RConn1
  Tooth 8/RConn1 -- tooth6/RConn1
  Tooth 6/RConn1 -- tooth7/RConn1
  Tooth 9/RConn1 -- tooth9/RConn1
  Tooth 7/RConn1 -- tooth8/RConn1
  Array Connection/RConn1 -- Magnetic Rotor/LConn3
  Array Connection1/RConn1 -- Magnetic Rotor/RConn1
  Array Connection1/LConn2 -- Array Connection1/LConn1 -- Array Connection1/LConn3 -- Array Connection1/LConn4 -- Magnetic Reference/LConn1 -- Array Connection1/LConn5 -- Array Connection1/LConn6 -- Array Connection1/LConn7 -- Array Connection1/LConn9 -- Array Connection1/LConn8

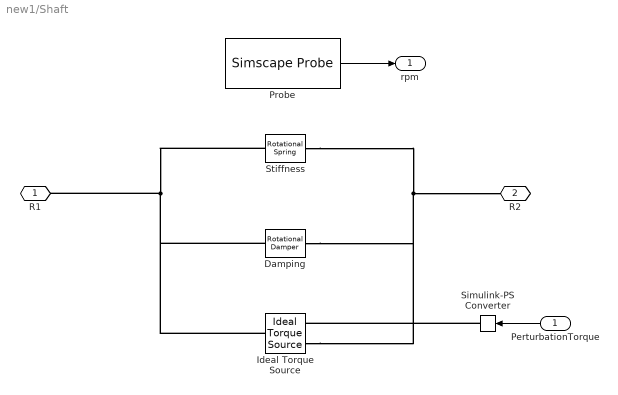
== system new1/Shaft ==
  PerturbationTorque : Inport
  Damping : fl_lib/Mechanical/Rotational Elements/Rotational Damper  D=ShaftDamping N*m*s/rad  w_specify=off  w_priority=None  w=0 rad/s  w_nominal_specify=off  w_nominal_value=1  w_nominal_unit=rad/s  t_specify=off  t_priority=None  t=0 N*m  t_nominal_specify=off  t_nominal_value=1  t_nominal_unit=N*m
  Ideal Torque Source : fl_lib/Mechanical/Mechanical Sources/Ideal Torque Source
  Probe : SimscapeProbe  BoundBlock=225  Variables="{\"R.w\":{\"Probing\":\"ON\"}}"
  Simulink-PS Converter : nesl_utility/Simulink-PS Converter  PhysicalDomain=network_engine_domain  SubClassName=ps_input  LeftPortType=input  RightPortType=output  PseudoPeriodic=off  Frequencies=[]  NoiseDistribution=none  NoiseParameters=[]  Unit=N*m  AffineConversion=off  FilteringAndDerivatives=provide  SimscapeFilterOrder=1  InputFilterTimeConstant=0.001  UdotUserProvided=0
  Stiffness : fl_lib/Mechanical/Rotational Elements/Rotational Spring  spr_rate=ShaftStiffness N*m/rad  w_specify=off  w_priority=None  w=0 rad/s  w_nominal_specify=off  w_nominal_value=1  w_nominal_unit=rad/s  t_specify=off  t_priority=None  t=0 N*m  t_nominal_specify=off  t_nominal_value=1  t_nominal_unit=N*m  phi_specify=on  phi_priority=High  phi=0 rad  phi_nominal_specify=off  phi_nominal_value=1  phi_nominal_unit=rad
  R1 : PMIOPort  Side=Left
  R2 : PMIOPort  Port=2  Side=Right
  rpm : Outport
  wires:
  PerturbationTorque/1 -> Simulink-PS Converter/1
  Probe/1 -> rpm/1
  connections:
  Stiffness/RConn1 -- Ideal Torque Source/RConn2 -- Damping/RConn1 -- R2/RConn1
  Stiffness/LConn1 -- Ideal Torque Source/LConn1 -- Damping/LConn1 -- R1/RConn1
  Simulink-PS Converter/RConn1 -- Ideal Torque Source/RConn1

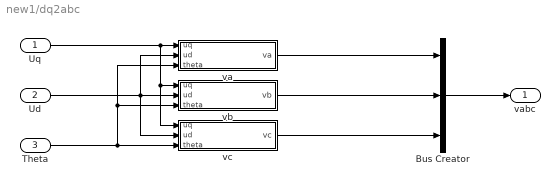
== system new1/dq2abc ==
  Uq : Inport
  Ud : Inport  Port=2
  Theta : Inport  Port=3
  Bus Creator : BusCreator  Inputs=3
  va : Subsystem
  vb : Subsystem
  vc : Subsystem
  vabc : Outport  VectorParamsAs1DForOutWhenUnconnected=off
  wires:
  vb/1(vb) -> Bus Creator/2
  Ud/1 -> va/2(ud), vb/2(ud), vc/2(ud)
  Uq/1 -> vc/1(uq), vb/1(uq), va/1(uq)
  va/1(va) -> Bus Creator/1
  Theta/1 -> va/3(theta), vb/3(theta), vc/3(theta)
  vc/1(vc) -> Bus Creator/3
  Bus Creator/1 -> vabc/1

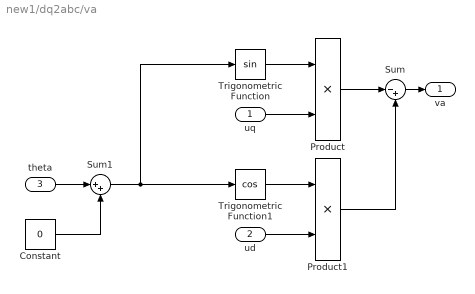
== system new1/dq2abc/va ==
  uq : Inport
  ud : Inport  Port=2
  theta : Inport  Port=3
  Constant : Constant  Value=0
  Product : Product
  Product1 : Product
  Sum : Sum  Inputs=|-+
  Sum1 : Sum  Inputs=|++
  Trigonometric Function : Trigonometry
  Trigonometric Function1 : Trigonometry  Operator=cos
  va : Outport  VectorParamsAs1DForOutWhenUnconnected=off
  wires:
  Product1/1 -> Sum/2
  Product/1 -> Sum/1
  ud/1 -> Product1/2
  Trigonometric Function/1 -> Product/1
  Trigonometric Function1/1 -> Product1/1
  Sum/1 -> va/1
  uq/1 -> Product/2
  Constant/1 -> Sum1/2
  theta/1 -> Sum1/1
  Sum1/1 -> Trigonometric Function1/1, Trigonometric Function/1

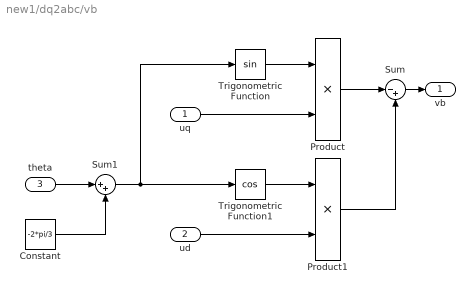
== system new1/dq2abc/vb ==
  uq : Inport
  ud : Inport  Port=2
  theta : Inport  Port=3
  Constant : Constant  Value=-2*pi/3
  Product : Product
  Product1 : Product
  Sum : Sum  Inputs=|-+
  Sum1 : Sum  Inputs=|++
  Trigonometric Function : Trigonometry
  Trigonometric Function1 : Trigonometry  Operator=cos
  vb : Outport  VectorParamsAs1DForOutWhenUnconnected=off
  wires:
  Product1/1 -> Sum/2
  Product/1 -> Sum/1
  ud/1 -> Product1/2
  Trigonometric Function/1 -> Product/1
  Trigonometric Function1/1 -> Product1/1
  Sum/1 -> vb/1
  uq/1 -> Product/2
  Constant/1 -> Sum1/2
  theta/1 -> Sum1/1
  Sum1/1 -> Trigonometric Function1/1, Trigonometric Function/1

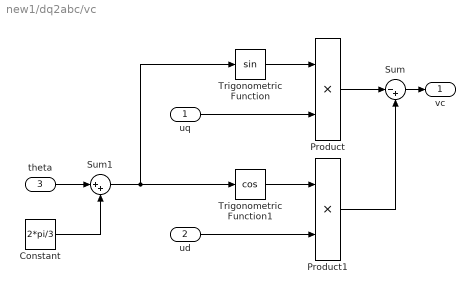
== system new1/dq2abc/vc ==
  uq : Inport
  ud : Inport  Port=2
  theta : Inport  Port=3
  Constant : Constant  Value=2*pi/3
  Product : Product
  Product1 : Product
  Sum : Sum  Inputs=|-+
  Sum1 : Sum  Inputs=|++
  Trigonometric Function : Trigonometry
  Trigonometric Function1 : Trigonometry  Operator=cos
  vc : Outport  VectorParamsAs1DForOutWhenUnconnected=off
  wires:
  Product1/1 -> Sum/2
  Product/1 -> Sum/1
  ud/1 -> Product1/2
  Trigonometric Function/1 -> Product/1
  Trigonometric Function1/1 -> Product1/1
  Sum/1 -> vc/1
  uq/1 -> Product/2
  Constant/1 -> Sum1/2
  theta/1 -> Sum1/1
  Sum1/1 -> Trigonometric Function1/1, Trigonometric Function/1
